simulink model "SSresonant"  (R2021a)
settings: Solver=ode45  StartTime=0.0  StopTime=5  FixedStep=0.0001  RelTol=1e-3
values from neighbouring files (symbols this model uses):
  Beq = 1.067548701517996e-06    (= 1.06754870152e-06)    [load_params_resonantLoad.m]
  den_B = [mld.Jb, mld.Bb]    [load_params_resonantLoad.m]
  H_den = [1, 2*H_damp*H_wc, H_wc^2]    [SS_LRQ_commonStart.m]
  H_num = [H_wc^2, 0]    [SS_LRQ_commonStart.m]
  Jeq = mot.J + mld.Jh/gbox.N^2    [load_params_resonantLoad.m]
  K = lqry(sysG,1,r)    [LQR_code_1to4.m]    (also in LQR_code_5to8.m = zeros(1,dimA); SSresonant_code.m = place(A, B, p))
  K_robust = zeros(1,dimA)    [LQR_code_1to4.m]    (also in LQR_code_5to8.m = [Ke(2) Ke(3) Ke(4) Ke(5)]; SSresonant_code.m = [Ke(2) Ke(3) Ke(4) Ke(5)])
  Ki_robust = 0    [LQR_code_1to4.m]    (also in LQR_code_5to8.m = Ke(1); SSresonant_code.m = Ke(1))
  Nu = Nxu(dimA+1)    [SS_LRQ_commonStart.m]
  Nx = [Nxu(1); Nxu(2); Nxu(3); Nxu(4)]    [SS_LRQ_commonStart.m]
  rads2rpm = 60/2/pi    (= 9.54929658551)    [load_params_resonantLoad.m]
  Req = mot.R + sens.curr.Rs    [load_params_resonantLoad.m]
  tau_sf = 0.012480599355650    (= 0.0124805993556)    [load_params_resonantLoad.m]
  Ts = 0.001    [PIDresonant_code.m]    (also in SS_LRQ_commonStart.m)
undefined symbols (not defined in the file or in its folder): daq, DiscIntNeverNeededParam, drv, gbox, mld, mot, sens
libraries: simulink x2
settings Model: Creator=giorgiadisaro  LastModifiedBy=utente-A
settings SolverCC: AlgebraicLoopSolver=TrustRegion
settings DebuggingCC: SFMachineParentedDataDiag=warning

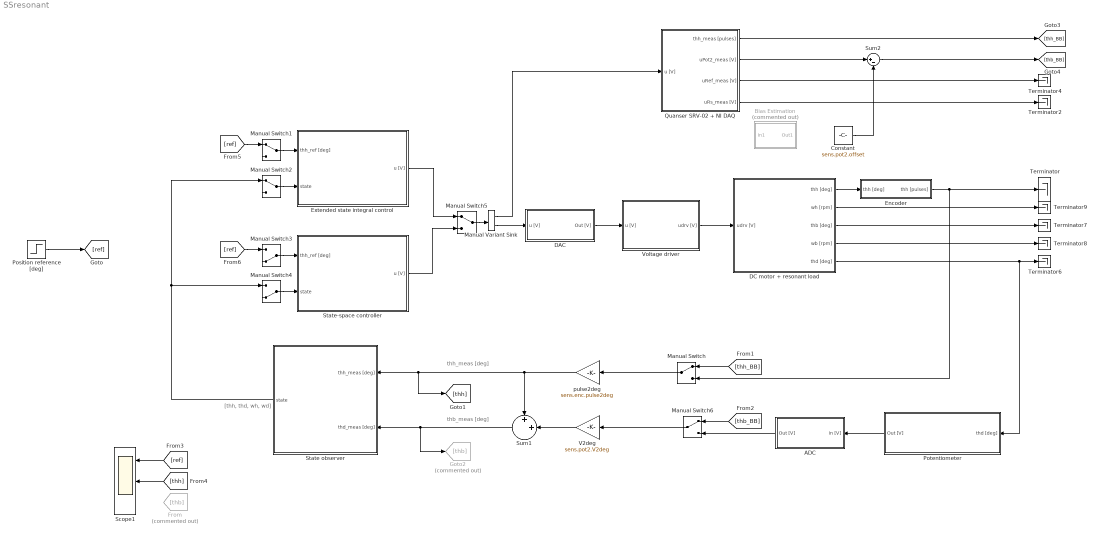
== system SSresonant ==
  note: [thh, thd, wh, wd]
  note: thh_meas [deg]
  note: thb_meas [deg]
  ADC : Subsystem
  Bias Estimation : Subsystem  Commented=on
  Constant : Constant  Value=sens.pot2.offset
  DAC : Subsystem
  DC motor + resonant load : Subsystem
  Encoder : Subsystem
  Extended state integral control : Subsystem
  From : From  Commented=on  GotoTag=thb
  Goto2 : Goto  Commented=on  GotoTag=thb
  Manual Variant Sink : simulink/Signal Routing/Manual Variant Sink  NumChoices=2  LabelModeActiveChoice=V_1
  Manual Switch{,1..2,5..6} (5 alike) : ManualSwitch
  Manual Switch3 : ManualSwitch  CurrentSetting=0
  Manual Switch4 : ManualSwitch  CurrentSetting=0
  Position reference [deg] : Step  After=50  SampleTime=0
  Potentiometer : Subsystem
  Quanser SRV-02 + NI DAQ : Subsystem  mask(Quanser SRV-02 (with resonant load) + NI DAQ){Ts=Ts, fricType=Karnopp, lockShaft=off, beamInitPos=10}
      mask prompts: Ts "NI DAQ Sample Time:"; fricType "Friction model"; lockShaft "Lock motor shaft"; beamInitPos "Beam initial position [deg]:"
      mask help: Quanser SRV-02 (with resonant load) + NI DAQ model.
      mask init:
      | %%
      | % Riccardo Antonello (riccardo.antonello@unipd.it)
      | %
      | % April 28, 2020
      | %
      | % Dept. of Information Engineering, University of Padova
      | %
      | 
      | %%  Conversion gains
      | deg2rad = pi/180;                   %   [deg]   -> [rad]
      | rad2deg = 180/pi;                   %   [rad]   -> [deg]
      | 
      | 
      | %%  Sensors data
      | 
      | %   shunt resistor
      | sens.curr.Rs = 0.5;   
      | 
      | %   Hewlett-Packard HEDS-5540#A06 optical encoder
      | sens.enc.ppr = 500*4;                                                   %   pulses per rotation
      | sens.enc.pulse2deg = 360/sens.enc.ppr;                                  %   [pulses] -> [deg]
      | sens.enc.pulse2rad = 2*pi/sens.enc.ppr;                                 %   [pulses] -> [rad]
      | sens.enc.deg2pulse = sens.enc.ppr/360;                                  %   [deg] -> [pulses]
      | sens.enc.rad2pulse = sens.enc.ppr/2/pi;                                 %   [rad] -> [pulses]
      | 
      | %   potentiometer 2 (Spectrol 357-0-0-103) - installed on hub
      | sens.pot2.range.R      = 10e3;                                          %   ohmic value range 
      | sens.pot2.range.V      = 5;                                             %   voltage range
      | sens.pot2.range.th_deg = 340;                                           %   angle range [deg]
      | sens.pot2.range.th     = sens.pot2.range.th_deg * deg2rad;              %   angle range [rad]                           
      | sens.pot2.deg2V        = sens.pot2.range.V / sens.pot2.range.th_deg;    %   sensitivity [V/deg]
      | sens.pot2.rad2V        = sens.pot2.range.V / sens.pot2.range.th;        %   sensitivity [V/rad]
      | sens.pot2.V2deg        = 1/sens.pot2.deg2V;                             %   conversion gain [V] -> [deg]
      | sens.pot2.V2rad        = 1/sens.pot2.rad2V;                             %   conversion gain [V] -> [rad]
      | sens.pot2.noise.var    = 3.5e-7;                                        %   out noise variance [V^2]
      | 
      | 
      | %%  Data acquisition board (daq) data
      | 
      | %   NI PCI-6221 DAC data
      | daq.dac.bits = 16;                                  %   resolution (bits)
      | daq.dac.fs   = 10;                                  %   full scale 
      | daq.dac.q    = 2*daq.dac.fs/(2^daq.dac.bits-1);     %	quantization
      | 
      | %   NI PCI-6221 ADC data
      | daq.adc.bits = 16;                                  %   resolution (bits)
      | daq.adc.fs   = 10;                                  %   full scale (as set in SLDRT Analog Input block)
      | daq.adc.q    = 2*daq.adc.fs/(2^daq.adc.bits-1);     %   quantization   
      | 
      | 
      | %%  Set beam initial position
      | % SRV02Handle = find_system(gcb, ...
      | %     'LookUnderMasks', 'on', ...
      | %     'FindAll', 'on', ...
      | %     'FollowLinks', 'on', ...
      | %     'SearchDepth', '1', ...
      | %     'BlockType', 'ModelReference', ...
      | %     'Name', 'Quanser SRV-02');
      | %
      | % %get_param(SRV02Handle, 'InstanceParameters')
      | % InstanceParams = get_param(SRV02Handle, 'InstanceParameters');
      | % for k = 1:length(InstanceParams)
      | %     if strcmp(InstanceParams(k).Name, 'thb0')
      | %         if lockShaft
      | %             InstanceParams(k).Value = sprintf('%f', beamInitPos);
      | %         else
      | %             InstanceParams(k).Value = sprintf('%f', 0);    
      | %         end
      | %         set_param(SRV02Handle, 'InstanceParameters', InstanceParams);
      | %         break;
      | %     end
      | % end
      | 
      | if lockShaft
      |     thb0 = beamInitPos;
      | else
      |     thb0 = 0;    
      | end
      | 
      | 
      | %%  Mask initialization
      | if lockShaft
      |     
      |     %   find Inport handle
      |     InPortHandle = find_system(gcb, ...
      |         'LookUnderMasks', 'on', ...
      |         'FindAll', 'on', ...
      |         'FollowLinks', 'on', ...
      |         'SearchDepth', '1', ...
      |         'BlockType', 'Inport', ...
      |         'Name', 'u [V]');
      |     
      |     if ~isempty(InPortHandle)
      |     
      |         %   find DAC handle
      |         DACHandle = find_system(gcb, ...
      |             'LookUnderMasks', 'on', ...
      |             'FindAll', 'on', ...
      |             'FollowLinks', 'on', ...
      |             'SearchDepth', '1', ...
      |             'BlockType', 'SubSystem', ...
      |             'Name', 'DAC');  
      | 
      |         %   remove Inport output connection   
      |         InportConn = get_param(InPortHandle, 'PortConnectivity');
      |         delete_line(gcb, InportConn.Position);
      | 
      |         %   remove Inport block
      |         delete_block(InPortHandle);
      | 
      |         %   add Constant block
      |         ConstantHandle = add_block( ...
      |             'simulink/Sources/Constant', [gcb, '/u [V]'], ...
      |             'Position', [20   -37    50   -23], ...
      |             'Value', '0');
      | 
      |         %   connect Constant to DAC block
      |         DACPortHandles = get_param(DACHandle, 'PortHandles');
      |         ConstantPortHandles = get_param(ConstantHandle, 'PortHandles');
      |         add_line(gcb, ConstantPortHandles.Outport(1), DACPortHandles.Inport(1));
      |     
      |     end
      |     
      | else
      |     
      |     %   find Constant handle
      |     ConstantHandle = find_system(gcb, ...
      |         'LookUnderMasks', 'on', ...
      |         'FindAll', 'on', ...
      |         'FollowLinks', 'on', ...
      |         'SearchDepth', '1', ...
      |         'BlockType', 'Constant', ...
      |         'Name', 'u [V]');
      |     
      |     if ~isempty(ConstantHandle)
      |     
      |         %   find DAC handle
      |         DACHandle = find_system(gcb, ...
      |             'LookUnderMasks', 'on', ...
      |             'FindAll', 'on', ...
      |             'FollowLinks', 'on', ...
      |             'SearchDepth', '1', ...
      |             'BlockType', 'SubSystem', ...
      |             'Name', 'DAC');  
      |  
      |         %   remove Constant output connection   
      |         ConstantConn = get_param(ConstantHandle, 'PortConnectivity');
      |         delete_line(gcb, ConstantConn.Position);
      | 
      |         %   remove Inport block
      |         delete_block(ConstantHandle);   
      | 
      |         %   add Inport block
      |         InportHandle = add_block( ...
      |             'simulink/Sources/In1', [gcb, '/u [V]'], ...
      |             'Position', [20   -37    50   -23], ...
      |             'Port', '1');
      | 
      |         %   connect Constant to DAC block
      |         DACPortHandles = get_param(DACHandle, 'PortHandles');
      |         InportPortHandles = get_param(InportHandle, 'PortHandles');
      |         add_line(gcb, InportPortHandles.Outport(1), DACPortHandles.Inport(1));
      |     
      |      end
      |     
      | end
      mask Help:
      | Riccardo Antonello (antonello@dei.unipd.it)
      | 
      | April 28, 2020
      | 
      | Dept. of Information Engineering, University of Padova
      mask TypeOptions fricType: Coulomb + viscous | Karnopp
      mask Callback lockShaft:
      | %   get status of check box
      | lockShaft = get_param(gcb, 'lockShaft');
      | 
      | %   get current value of MaskVisibilities property
      | maskVisibilities = get_param(gcb, 'MaskVisibilities');
      | 
      | %   set visibility of the dialog box element
      | if strcmp(lockShaft, 'on')
      |     maskVisibilities{4} = 'on';
      | else
      |     maskVisibilities{4} = 'off';
      | end
      | 
      | % Set the 'MaskVisibilities' property for each parameter in mask
      | set_param( gcb, 'MaskVisibilities', maskVisibilities);
  Scope1 : Scope  NumInputPorts=3
  State observer : Subsystem
  State-space controller : Subsystem
  Sum1 : Sum  Inputs=++|
  Sum2 : Sum  Inputs=|+-
  Terminator{,2,4,6..9} (7 alike) : Terminator
  V2deg : Gain  Gain=sens.pot2.V2deg
  Voltage driver : Subsystem
  pulse2deg : Gain  Gain=sens.enc.pulse2deg
  wires:
  Manual Switch5/1 -> Manual Variant Sink/1
  Position reference [deg]/1 -> [ref]
  Extended state integral control/1(u [V]) -> Manual Switch5/1
  State-space controller/1(u [V]) -> Manual Switch5/2
  Manual Switch1/1 -> Extended state integral control/1(thh_ref [deg])
  Manual Switch2/1 -> Extended state integral control/2(state)
  Manual Switch3/1 -> State-space controller/1(thh_ref [deg])
  Manual Switch4/1 -> State-space controller/2(state)
  State observer/1(state) -> Manual Switch4/1, Manual Switch2/1
  [thh_BB] -> Manual Switch/1
  ADC/1(Out [V]) -> Manual Switch6/2
  Sum1/1 -> State observer/2(thd_meas [deg]), Goto2/1
  Voltage driver/1(udrv [V]) -> DC motor + resonant load/1(udrv [V])
  [thb_BB] -> Manual Switch6/1
  V2deg/1 -> Sum1/2
  DC motor + resonant load/2(wh [rpm]) -> Terminator9/1
  DC motor + resonant load/3(thb [deg]) -> Terminator7/1
  Potentiometer/1(Out [V]) -> ADC/1(in [V])
  DC motor + resonant load/5(thd [deg]) -> Potentiometer/1(thd [deg]), Terminator6/1
  DC motor + resonant load/4(wb [rpm]) -> Terminator8/1
  pulse2deg/1 -> Sum1/1, [thh], State observer/1(thh_meas [deg])
  DAC/1(Out [V]) -> Voltage driver/1(u [V])
  DC motor + resonant load/1("thh [deg] ") -> Encoder/1("thh [deg] ")
  Manual Variant Sink/1 -> Quanser SRV-02 + NI DAQ/1(u [V])
  Manual Switch/1 -> pulse2deg/1
  Quanser SRV-02 + NI DAQ/3(uRef_meas [V]) -> Terminator4/1
  Encoder/1(thh [pulses]) -> Manual Switch/2, Terminator/1
  Quanser SRV-02 + NI DAQ/2(uPot2_meas [V]) -> Sum2/1
  Manual Switch6/1 -> V2deg/1
  Quanser SRV-02 + NI DAQ/4(uRs_meas [V]) -> Terminator2/1
  Quanser SRV-02 + NI DAQ/1(thh_meas [pulses]) -> [thh_BB]
  Manual Variant Sink/2 -> DAC/1(u [V])
  [thh] -> Scope1/2
  [ref] -> Scope1/1
  Constant/1 -> Sum2/2
  Sum2/1 -> [thb_BB]
  [ref] -> Manual Switch1/1
  [ref] -> Manual Switch3/1

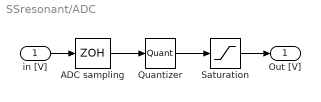
== system SSresonant/ADC ==
  in [V] : Inport
  ADC sampling : ZeroOrderHold  SampleTime=Ts
  Quantizer : Quantizer  QuantizationInterval=daq.adc.q
  Saturation : Saturate  UpperLimit=daq.adc.fs  LowerLimit=-daq.adc.fs
  Out [V] : Outport
  wires:
  in [V]/1 -> ADC sampling/1
  ADC sampling/1 -> Quantizer/1
  Quantizer/1 -> Saturation/1
  Saturation/1 -> Out [V]/1

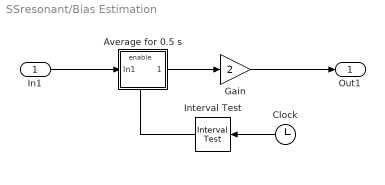
== system SSresonant/Bias Estimation ==
  In1 : Inport
  Average for 0.5 s : Subsystem
  Clock : Clock
  Gain : Gain  Gain=2
  Interval Test : simulink/Logic and Bit Operations/Interval Test  IntervalClosedRight=on  uplimit=0.7  IntervalClosedLeft=on  lowlimit=0.2  OutDataTypeStr=boolean
  Out1 : Outport
  wires:
  Gain/1 -> Out1/1
  Average for 0.5 s/1(Out1) -> Gain/1
  Clock/1 -> Interval Test/1
  In1/1 -> Average for 0.5 s/1(In1)
  Interval Test/1 -> Average for 0.5 s/Enable

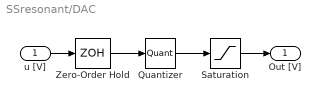
== system SSresonant/DAC ==
  u [V] : Inport
  Quantizer : Quantizer  QuantizationInterval=20/(2^16-1)
  Saturation : Saturate  UpperLimit=10  LowerLimit=-10
  Zero-Order Hold : ZeroOrderHold  SampleTime=Ts
  Out [V] : Outport
  wires:
  u [V]/1 -> Zero-Order Hold/1
  Zero-Order Hold/1 -> Quantizer/1
  Quantizer/1 -> Saturation/1
  Saturation/1 -> Out [V]/1

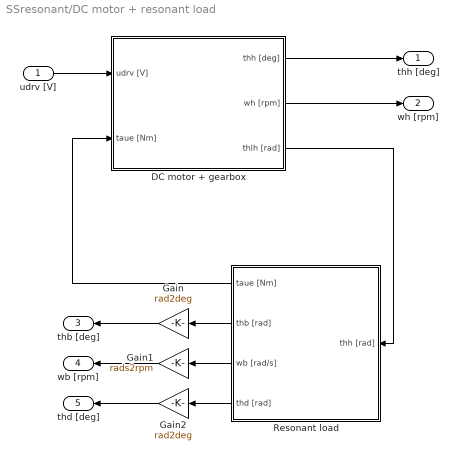
== system SSresonant/DC motor + resonant load ==
  udrv [V] : Inport
  DC motor + gearbox : Subsystem
  Gain : Gain  Gain=rad2deg
  Gain1 : Gain  Gain=rads2rpm
  Gain2 : Gain  Gain=rad2deg
  Resonant load : Subsystem
  "thh [deg] " : Outport
  wh [rpm] : Outport  Port=2
  thb [deg] : Outport  Port=3
  wb [rpm] : Outport  Port=4
  thd [deg] : Outport  Port=5
  wires:
  DC motor + gearbox/3(thlh [rad]) -> Resonant load/1(thh [rad])
  DC motor + gearbox/1("thh [deg] ") -> "thh [deg] "/1
  Resonant load/1(taue [Nm]) -> DC motor + gearbox/2(taue [Nm])
  udrv [V]/1 -> DC motor + gearbox/1(udrv [V])
  DC motor + gearbox/2(wh [rpm]) -> wh [rpm]/1
  Resonant load/2(thb [rad]) -> Gain/1
  Gain/1 -> thb [deg]/1
  Gain1/1 -> wb [rpm]/1
  Resonant load/3(wb [rad/s]) -> Gain1/1
  Resonant load/4(thd [rad]) -> Gain2/1
  Gain2/1 -> thd [deg]/1

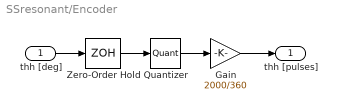
== system SSresonant/Encoder ==
  "thh [deg] " : Inport
  Gain : Gain  Gain=2000/360
  Quantizer : Quantizer  QuantizationInterval=360/(500*4)
  Zero-Order Hold : ZeroOrderHold  SampleTime=Ts
  thh [pulses] : Outport
  wires:
  "thh [deg] "/1 -> Zero-Order Hold/1
  Zero-Order Hold/1 -> Quantizer/1
  Quantizer/1 -> Gain/1
  Gain/1 -> thh [pulses]/1

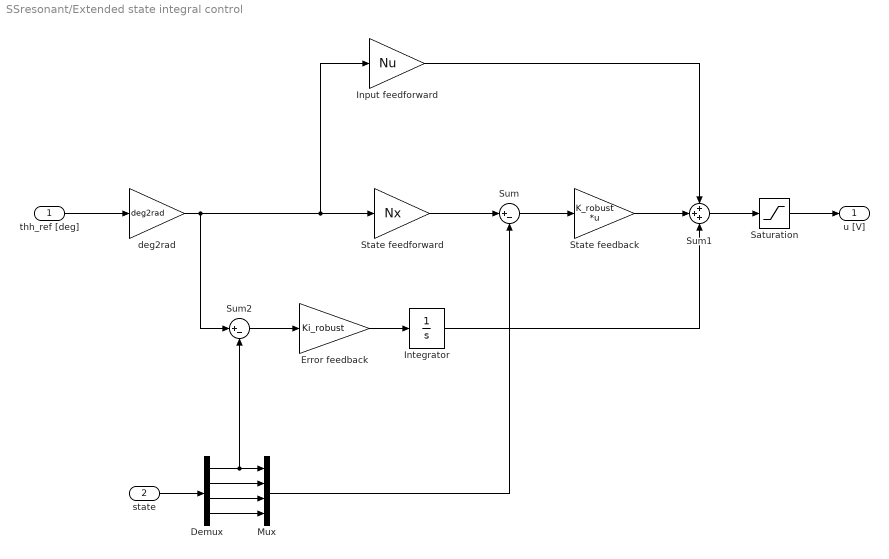
== system SSresonant/Extended state integral control ==
  thh_ref [deg] : Inport
  state : Inport  Port=2
  Demux : Demux
  Error feedback : Gain  Gain=Ki_robust
  Input feedforward : Gain  Gain=Nu
  Integrator : Integrator
  Mux : Mux
  Saturation : Saturate  UpperLimit=12  LowerLimit=-12
  State feedback : Gain  Gain=K_robust  Multiplication=Matrix(K*u) (u vector)
  State feedforward : Gain  Gain=Nx
  Sum : Sum  Inputs=|+-
  Sum1 : Sum  Inputs=+++
  Sum2 : Sum  Inputs=|+-
  deg2rad : Gain  Gain=deg2rad
  u [V] : Outport
  wires:
  Saturation/1 -> u [V]/1
  deg2rad/1 -> State feedforward/1, Input feedforward/1, Sum2/1
  Sum/1 -> State feedback/1
  thh_ref [deg]/1 -> deg2rad/1
  State feedforward/1 -> Sum/1
  State feedback/1 -> Sum1/2
  Input feedforward/1 -> Sum1/1
  Sum1/1 -> Saturation/1
  Sum2/1 -> Error feedback/1
  Error feedback/1 -> Integrator/1
  Integrator/1 -> Sum1/3
  Demux/1 -> Sum2/2, Mux/1
  Demux/2 -> Mux/2
  Demux/3 -> Mux/3
  Demux/4 -> Mux/4
  state/1 -> Demux/1
  Mux/1 -> Sum/2

== system SSresonant/Potentiometer ==
  thd [deg] : Inport
  Gain : Gain  Gain=sens.pot2.deg2V
  Sum : Sum  Inputs=|++
  sensor output noise [V] : RandomNumber  Variance=sens.pot2.noise.var  SampleTime=Ts
  Out [V] : Outport
  wires:
  thd [deg]/1 -> Gain/1
  Gain/1 -> Sum/1
  Sum/1 -> Out [V]/1
  sensor output noise [V]/1 -> Sum/2

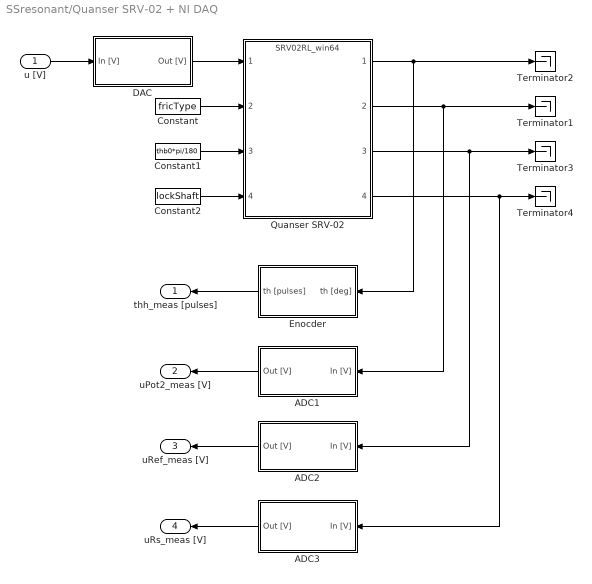
== system SSresonant/Quanser SRV-02 + NI DAQ ==
  u [V] : Inport
  ADC1 : Subsystem
  ADC2 : Subsystem
  ADC3 : Subsystem
  Constant : Constant  Value=fricType
  Constant1 : Constant  Value=thb0*pi/180  SampleTime=Inf
  Constant2 : Constant  Value=lockShaft  SampleTime=Inf
  DAC : Subsystem
  Enocder : Subsystem
  Quanser SRV-02 : ModelReference  ModelNameDialog=SRV02RL_win64.slxp  ModelReferenceVersion=1.76  CopyOfModelProtected=on
  Terminator{1..4} (4 alike) : Terminator
  thh_meas [pulses] : Outport
  uPot2_meas [V] : Outport  Port=2
  uRef_meas [V] : Outport  Port=3
  uRs_meas [V] : Outport  Port=4
  wires:
  Enocder/1(th [pulses]) -> thh_meas [pulses]/1
  ADC3/1(Out [V]) -> uRs_meas [V]/1
  DAC/1(Out [V]) -> Quanser SRV-02/1
  Quanser SRV-02/2 -> ADC1/1(In [V]), Terminator1/1
  Quanser SRV-02/1 -> Terminator2/1, Enocder/1(th [deg])
  Constant/1 -> Quanser SRV-02/2
  Quanser SRV-02/3 -> ADC2/1(In [V]), Terminator3/1
  ADC1/1(Out [V]) -> uPot2_meas [V]/1
  Constant1/1 -> Quanser SRV-02/3
  Constant2/1 -> Quanser SRV-02/4
  Quanser SRV-02/4 -> ADC3/1(In [V]), Terminator4/1
  ADC2/1(Out [V]) -> uRef_meas [V]/1
  u [V]/1 -> DAC/1(In [V])

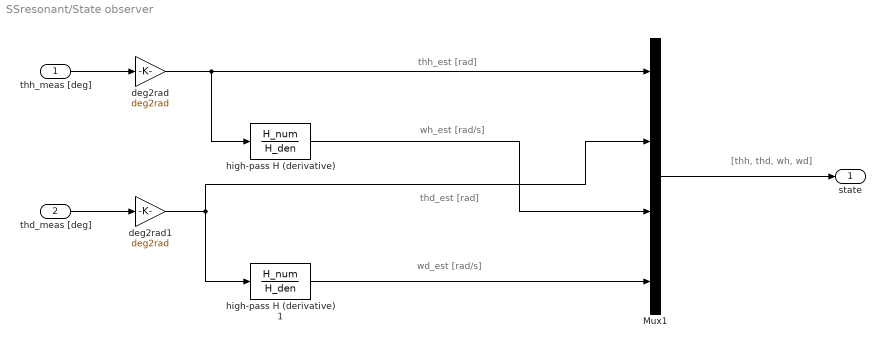
== system SSresonant/State observer ==
  note: [thh, thd, wh, wd]
  note: wd_est [rad/s]
  note: thd_est [rad]
  note: wh_est [rad/s]
  note: thh_est [rad]
  thh_meas [deg] : Inport
  thd_meas [deg] : Inport  Port=2
  Mux1 : Mux
  deg2rad : Gain  Gain=deg2rad
  deg2rad1 : Gain  Gain=deg2rad
  high-pass H (derivative) : TransferFcn  Numerator=H_num  Denominator=H_den
  high-pass H (derivative)1 : TransferFcn  Numerator=H_num  Denominator=H_den
  state : Outport
  wires:
  thd_meas [deg]/1 -> deg2rad1/1
  deg2rad1/1 -> high-pass H (derivative)1/1, Mux1/2
  deg2rad/1 -> Mux1/1, high-pass H (derivative)/1
  Mux1/1 -> state/1
  high-pass H (derivative)/1 -> Mux1/3
  thh_meas [deg]/1 -> deg2rad/1
  high-pass H (derivative)1/1 -> Mux1/4

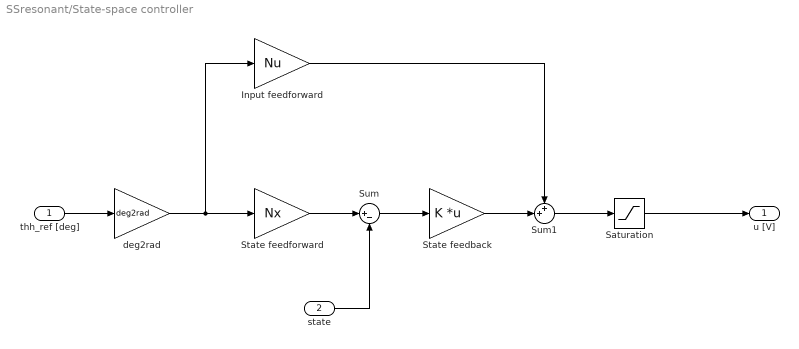
== system SSresonant/State-space controller ==
  thh_ref [deg] : Inport
  state : Inport  Port=2
  Input feedforward : Gain  Gain=Nu
  Saturation : Saturate  UpperLimit=12  LowerLimit=-12
  State feedback : Gain  Gain=K  Multiplication=Matrix(K*u) (u vector)
  State feedforward : Gain  Gain=Nx
  Sum : Sum  Inputs=|+-
  Sum1 : Sum  Inputs=++|
  deg2rad : Gain  Gain=deg2rad
  u [V] : Outport
  wires:
  Saturation/1 -> u [V]/1
  deg2rad/1 -> State feedforward/1, Input feedforward/1
  Sum/1 -> State feedback/1
  thh_ref [deg]/1 -> deg2rad/1
  State feedforward/1 -> Sum/1
  State feedback/1 -> Sum1/2
  Input feedforward/1 -> Sum1/1
  Sum1/1 -> Saturation/1
  state/1 -> Sum/2

== system SSresonant/Voltage driver ==
  u [V] : Inport
  Saturation : Saturate  UpperLimit=10  LowerLimit=-10
  Transfer Fcn : TransferFcn  Numerator=[drv.dcgain]  Denominator=[drv.Tc 1]
  udrv [V] : Outport
  wires:
  u [V]/1 -> Transfer Fcn/1
  Transfer Fcn/1 -> Saturation/1
  Saturation/1 -> udrv [V]/1

== system SSresonant/Bias Estimation/Average for 0.5 s ==
  In1 : Inport
  Enable : EnablePort
  Discrete-Time Integrator : DiscreteIntegrator  SampleTime=Ts  ICPrevOutput=DiscIntNeverNeededParam  ICPrevScaledInput=DiscIntNeverNeededParam
  Out1 : Outport
  wires:
  Discrete-Time Integrator/1 -> Out1/1
  In1/1 -> Discrete-Time Integrator/1

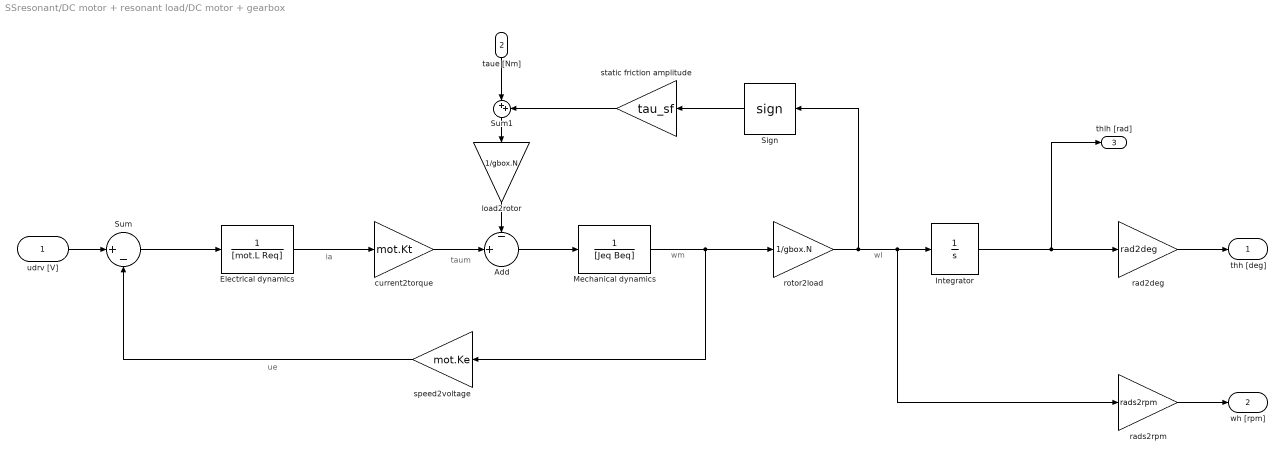
== system SSresonant/DC motor + resonant load/DC motor + gearbox ==
  note: wl
  note: wm
  note: ue
  note: taum
  note: ia
  udrv [V] : Inport
  taue [Nm] : Inport  Port=2
  Add : Sum  Inputs=-|+||
  Electrical dynamics : TransferFcn  Denominator=[mot.L Req]
  Integrator : Integrator
  Mechanical dynamics : TransferFcn  Denominator=[Jeq Beq]
  Sign : Signum  ZeroCross=off
  Sum : Sum  Inputs=|+-
  Sum1 : Sum  Inputs=|++
  current2torque : Gain  Gain=mot.Kt
  load2rotor : Gain  Gain=1/gbox.N
  rad2deg : Gain  Gain=rad2deg
  rads2rpm : Gain  Gain=rads2rpm
  rotor2load : Gain  Gain=1/gbox.N
  speed2voltage : Gain  Gain=mot.Ke
  static friction amplitude : Gain  Gain=tau_sf
  "thh [deg] " : Outport
  wh [rpm] : Outport  Port=2
  thlh [rad] : Outport  Port=3
  wires:
  udrv [V]/1 -> Sum/1
  Electrical dynamics/1 -> current2torque/1
  current2torque/1 -> Add/2
  load2rotor/1 -> Add/1
  Sign/1 -> static friction amplitude/1
  speed2voltage/1 -> Sum/2
  rad2deg/1 -> "thh [deg] "/1
  Add/1 -> Mechanical dynamics/1
  Mechanical dynamics/1 -> speed2voltage/1, rotor2load/1
  rads2rpm/1 -> wh [rpm]/1
  Sum/1 -> Electrical dynamics/1
  rotor2load/1 -> Sign/1, rads2rpm/1, Integrator/1
  Integrator/1 -> rad2deg/1, thlh [rad]/1
  Sum1/1 -> load2rotor/1
  static friction amplitude/1 -> Sum1/2
  taue [Nm]/1 -> Sum1/1

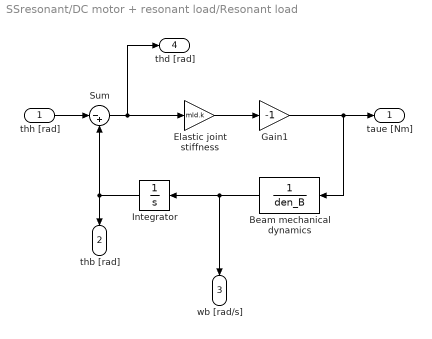
== system SSresonant/DC motor + resonant load/Resonant load ==
  thh [rad] : Inport
  Beam mechanical dynamics : TransferFcn  Denominator=den_B
  Elastic joint stiffness : Gain  Gain=mld.k
  Gain1 : Gain  Gain=-1
  Integrator : Integrator
  Sum : Sum  Inputs=|-+
  taue [Nm] : Outport
  thb [rad] : Outport  Port=2
  wb [rad/s] : Outport  Port=3
  thd [rad] : Outport  Port=4
  wires:
  thh [rad]/1 -> Sum/1
  Integrator/1 -> thb [rad]/1, Sum/2
  Beam mechanical dynamics/1 -> Integrator/1, wb [rad/s]/1
  Sum/1 -> Elastic joint stiffness/1, thd [rad]/1
  Elastic joint stiffness/1 -> Gain1/1
  Gain1/1 -> Beam mechanical dynamics/1, taue [Nm]/1

== system SSresonant/Quanser SRV-02 + NI DAQ/ADC1 ==
  In [V] : Inport
  ADC quantization : Quantizer  QuantizationInterval=daq.adc.q
  ADC sampling : ZeroOrderHold  SampleTime=Ts
  ADC saturation : Saturate  UpperLimit=daq.adc.fs  LowerLimit=-daq.adc.fs
  Out [V] : Outport
  wires:
  ADC saturation/1 -> Out [V]/1
  ADC sampling/1 -> ADC quantization/1
  In [V]/1 -> ADC sampling/1
  ADC quantization/1 -> ADC saturation/1

== system SSresonant/Quanser SRV-02 + NI DAQ/ADC2 ==
  In [V] : Inport
  ADC quantization : Quantizer  QuantizationInterval=daq.adc.q
  ADC sampling : ZeroOrderHold  SampleTime=Ts
  ADC saturation : Saturate  UpperLimit=daq.adc.fs  LowerLimit=-daq.adc.fs
  Out [V] : Outport
  wires:
  ADC quantization/1 -> ADC saturation/1
  In [V]/1 -> ADC sampling/1
  ADC sampling/1 -> ADC quantization/1
  ADC saturation/1 -> Out [V]/1

== system SSresonant/Quanser SRV-02 + NI DAQ/ADC3 ==
  In [V] : Inport
  Quantizer : Quantizer  QuantizationInterval=daq.adc.q
  Saturation : Saturate  UpperLimit=daq.adc.fs  LowerLimit=-daq.adc.fs
  Zero-Order Hold : ZeroOrderHold  SampleTime=Ts
  Out [V] : Outport
  wires:
  Saturation/1 -> Out [V]/1
  In [V]/1 -> Zero-Order Hold/1
  Quantizer/1 -> Saturation/1
  Zero-Order Hold/1 -> Quantizer/1

== system SSresonant/Quanser SRV-02 + NI DAQ/DAC ==
  In [V] : Inport
  Quantizer : Quantizer  QuantizationInterval=daq.dac.q
  Saturation : Saturate  UpperLimit=daq.dac.fs  LowerLimit=-daq.dac.fs
  Zero-Order Hold : ZeroOrderHold  SampleTime=Ts
  Out [V] : Outport
  wires:
  Quantizer/1 -> Saturation/1
  In [V]/1 -> Zero-Order Hold/1
  Zero-Order Hold/1 -> Quantizer/1
  Saturation/1 -> Out [V]/1

== system SSresonant/Quanser SRV-02 + NI DAQ/Enocder ==
  th [deg] : Inport
  Quantizer : Quantizer  QuantizationInterval=sens.enc.pulse2deg
  Zero-Order Hold : ZeroOrderHold  SampleTime=Ts
  deg2pulse : Gain  Gain=sens.enc.deg2pulse
  th [pulses] : Outport
  wires:
  Quantizer/1 -> deg2pulse/1
  th [deg]/1 -> Zero-Order Hold/1
  Zero-Order Hold/1 -> Quantizer/1
  deg2pulse/1 -> th [pulses]/1
